simulink model "RTinductionmotor"  (R2020b)
settings: Solver=VariableStepAuto  StartTime=0.0  StopTime=0.25  RelTol=1e-3
libraries: powerlib_meascontrol x1
settings Model: Creator=adam_  LastModifiedBy=adam_

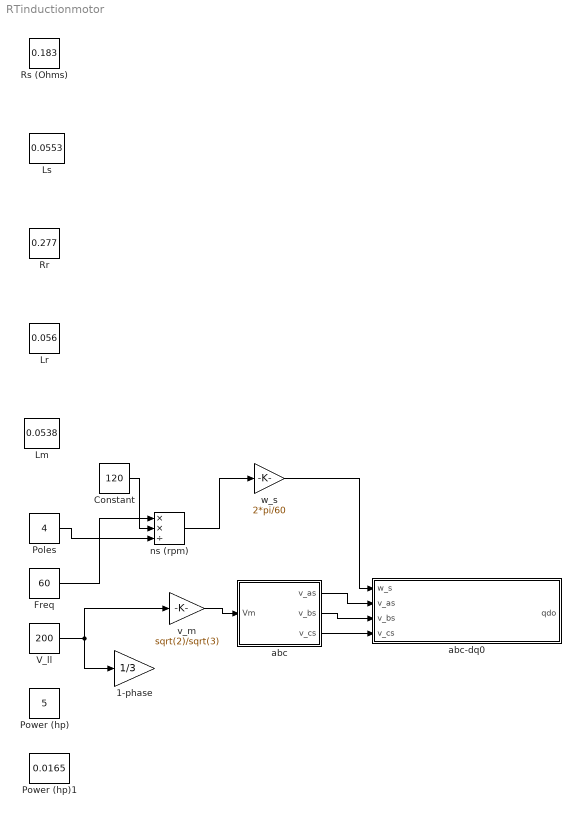
== system RTinductionmotor ==
  1-phase : Gain  Gain=1/3
  Constant : Constant  Value=120
  Freq : Constant  Value=60
  "Lm " : Constant  Value=0.0538
  Lr : Constant  Value=0.056
  "Ls " : Constant  Value=0.0553
  Poles : Constant  Value=4
  Power (hp) : Constant  Value=5
  Power (hp)1 : Constant  Value=0.0165
  "Rr " : Constant  Value=0.277
  Rs (Ohms) : Constant  Value=0.183
  V_ll : Constant  Value=200
  abc : Subsystem
  abc-dq0 : Subsystem
  ns (rpm) : Product  Inputs=**/
  v_m : Gain  Gain=sqrt(2)/sqrt(3)
  w_s : Gain  Gain=2*pi/60
  wires:
  V_ll/1 -> v_m/1, 1-phase/1
  Freq/1 -> ns (rpm)/1
  Poles/1 -> ns (rpm)/3
  Constant/1 -> ns (rpm)/2
  abc/1(v_as) -> abc-dq0/2(v_as)
  abc/2(v_bs) -> abc-dq0/3(v_bs)
  abc/3(v_cs) -> abc-dq0/4(v_cs)
  ns (rpm)/1 -> w_s/1
  w_s/1 -> abc-dq0/1(w_s)
  v_m/1 -> abc/1(Vm)

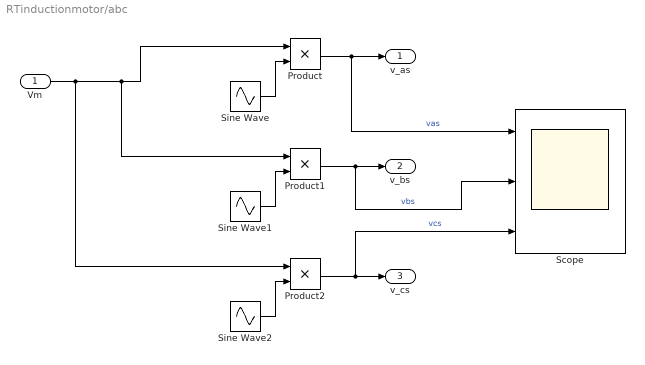
== system RTinductionmotor/abc ==
  Vm : Inport
  Product : Product
  Product1 : Product
  Product2 : Product
  Scope : Scope  NumInputPorts=3
  Sine Wave : Sin  Frequency=60*2*pi  SampleTime=0.0001  VectorParams1D=off
  Sine Wave1 : Sin  Frequency=60*2*pi  Phase=-2*pi/3  SampleTime=0.0001  VectorParams1D=off
  Sine Wave2 : Sin  Frequency=60*2*pi  Phase=2*pi/3  SampleTime=0.0001  VectorParams1D=off
  v_as : Outport
  v_bs : Outport  Port=2
  v_cs : Outport  Port=3
  wires:
  Sine Wave/1 -> Product/2
  Product/1 -> Scope/1, v_as/1  "vas"
  Product1/1 -> Scope/2, v_bs/1  "vbs"
  Sine Wave1/1 -> Product1/2
  Product2/1 -> Scope/3, v_cs/1  "vcs"
  Vm/1 -> Product2/1, Product1/1, Product/1
  Sine Wave2/1 -> Product2/2

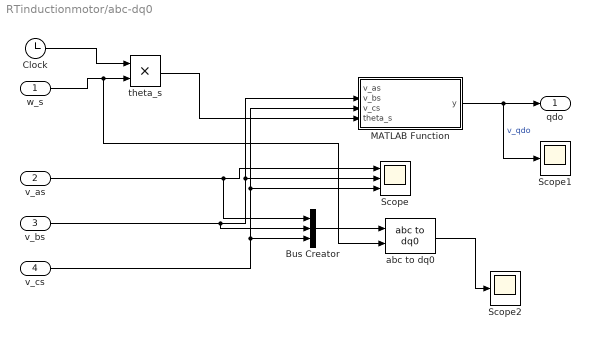
== system RTinductionmotor/abc-dq0 ==
  w_s : Inport
  v_as : Inport  Port=2
  v_bs : Inport  Port=3
  v_cs : Inport  Port=4
  Bus Creator : BusCreator  Inputs=3
  Clock : Clock
  MATLAB Function : MATLAB Function  TreatAsAtomicUnit=on
  Scope : Scope  NumInputPorts=3
  Scope1 : Scope
  Scope2 : Scope
  abc to dq0 : powerlib_meascontrol/Transformations/abc to dq0  Alignment=90 degrees behind phase A axis
  theta_s : Product
  qdo : Outport
  wires:
  v_as/1 -> Bus Creator/1, Scope/1
  v_cs/1 -> Bus Creator/3, Scope/3, MATLAB Function/3(v_cs)
  MATLAB Function/1(y) -> Scope1/1, qdo/1  "v_qdo"
  v_bs/1 -> Bus Creator/2, Scope/2, MATLAB Function/2(v_bs)
  w_s/1 -> abc to dq0/2, theta_s/2
  Clock/1 -> theta_s/1
  theta_s/1 -> MATLAB Function/4(theta_s)
  Bus Creator/1 -> abc to dq0/1
  abc to dq0/1 -> Scope2/1

== matlab function RTinductionmotor/abc-dq0/MATLAB Function ==
  data: v_as input; y output; v_bs input; v_cs input; theta_s input
function y = fcn(v_as, v_bs, v_cs, theta_s)
%#codegen
T_abc = 2/3 * ...
    [ cos(theta_s) cos(theta_s-(2*pi/3)) cos(theta_s + (2*pi/3));...
    sin(theta_s) sin(theta_s-(2*pi/3)) sin(theta_s + (2*pi/3));...
    1/2 1/2 1/2 ];
v_abc = [ v_as;v_bs;v_cs] ; 
v_qdo = T_abc * v_abc ;
y = v_qdo;
